simulink model "sys_sim_sen"  (R2021a)
settings: Solver=VariableStepAuto  StartTime=0.0  StopTime=30  RelTol=1e-3
settings Model: Creator=Suman  LastModifiedBy=Suman

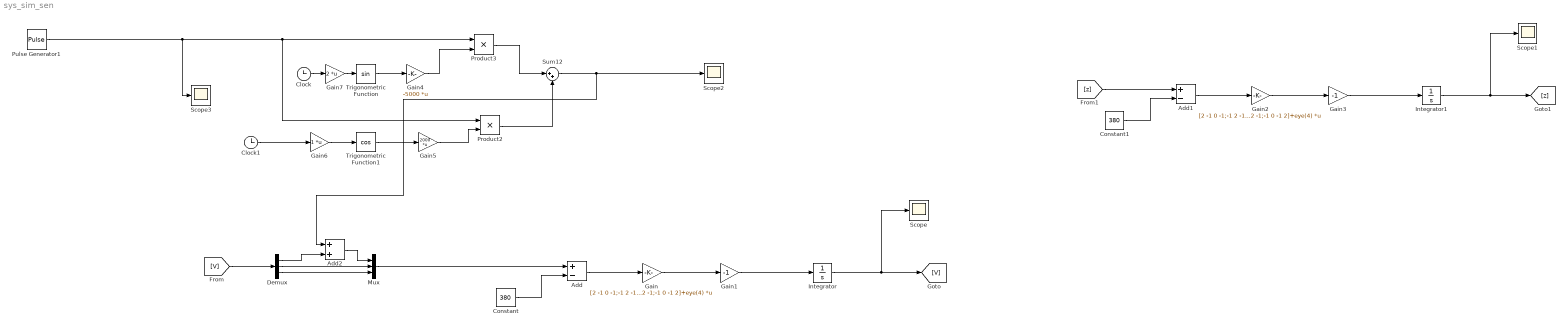
== system sys_sim_sen ==
  Add : Sum  Inputs=+-
  Add1 : Sum  Inputs=+-
  Add2 : Sum
  Clock : Clock
  Clock1 : Clock
  Constant : Constant  Value=380
  Constant1 : Constant  Value=380
  Demux : Demux  Outputs=3
  Gain : Gain  Gain=[2 -1 0 -1;-1 2 -1 0;0 -1 2 -1;-1 0 -1 2]+eye(4)  Multiplication=Matrix(K*u) (u vector)
  Gain1 : Gain  Gain=-1
  Gain2 : Gain  Gain=[2 -1 0 -1;-1 2 -1 0;0 -1 2 -1;-1 0 -1 2]+eye(4)  Multiplication=Matrix(K*u) (u vector)
  Gain3 : Gain  Gain=-1
  Gain4 : Gain  Gain=-5000  Multiplication=Matrix(K*u) (u vector)
  Gain5 : Gain  Gain=2000  Multiplication=Matrix(K*u) (u vector)
  Gain6 : Gain  Multiplication=Matrix(K*u) (u vector)
  Gain7 : Gain  Gain=2  Multiplication=Matrix(K*u) (u vector)
  Integrator : Integrator  InitialCondition="[287.1501 ; 145.6127 ; 240.0841 ;  42.5659]"
  Integrator1 : Integrator  InitialCondition="[287.1501 ; 145.6127 ; 240.0841 ;  42.5659]"
  Mux : Mux  Inputs=3
  Product2 : Product
  Product3 : Product
  Pulse Generator1 : DiscretePulseGenerator  PulseType=Time based  Period=30  PulseWidth=10  PhaseDelay=10
  Scope{,1..3} (4 alike) : Scope
  Sum12 : Sum  Inputs=|++
  Trigonometric Function : Trigonometry
  Trigonometric Function1 : Trigonometry  Operator=cos
  wires:
  Gain/1 -> Gain1/1
  Gain1/1 -> Integrator/1
  Integrator/1 -> Scope/1, [V]
  Add/1 -> Gain/1
  Constant/1 -> Add/2
  Add1/1 -> Gain2/1
  [z] -> Add1/1
  Constant1/1 -> Add1/2
  Integrator1/1 -> Scope1/1, [z]
  Gain2/1 -> Gain3/1
  Gain3/1 -> Integrator1/1
  Gain6/1 -> Trigonometric Function1/1
  Product2/1 -> Sum12/2
  Pulse Generator1/1 -> Scope3/1, Product2/1, Product3/1
  Sum12/1 -> Add2/1, Scope2/1
  Product3/1 -> Sum12/1
  Gain7/1 -> Trigonometric Function/1
  Clock/1 -> Gain7/1
  Clock1/1 -> Gain6/1
  Trigonometric Function1/1 -> Gain5/1
  Gain5/1 -> Product2/2
  Trigonometric Function/1 -> Gain4/1
  Gain4/1 -> Product3/2
  [V] -> Demux/1
  Demux/3 -> Mux/3
  Demux/2 -> Mux/2
  Demux/1 -> Add2/2
  Add2/1 -> Mux/1
  Mux/1 -> Add/1
